simulink library "AVE_Library"  (R2025b)
settings: Solver=VariableStepAuto  StartTime=0.0  StopTime=10.0  RelTol=1e-3
undefined symbols (not defined in the file or in its folder): DiscIntNeverNeededParam
libraries: simulink x44, etargetslib x18, $bdroot x13, GenericTarget x2
(part 4 of 5)

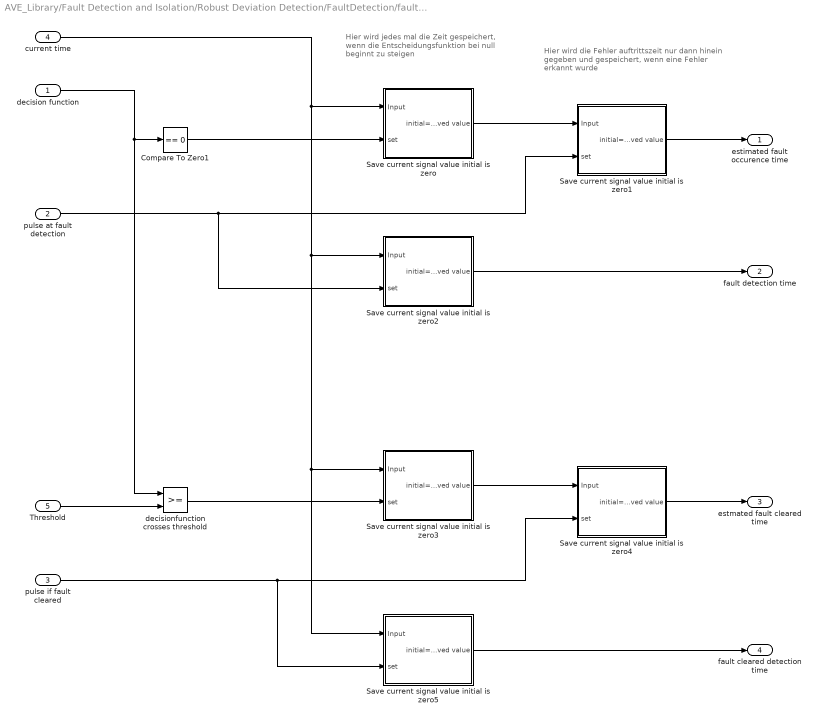
== system AVE_Library/Fault Detection and Isolation/Robust Deviation Detection/FaultDetection/fault occurence time3 ==
  note: Hier wird jedes mal die Zeit gespeichert,
      | wenn die Entscheidungsfunktion bei null
      | beginnt zu steigen
  note: Hier wird die Fehler auftrittszeit nur dann hinein
      | gegeben und gespeichert, wenn eine Fehler
      | erkannt wurde
  decision function : Inport
  pulse at fault detection : Inport  Port=2
  pulse if fault cleared : Inport  Port=3
  current time : Inport  Port=4
  Threshold : Inport  Port=5
  Compare To Zero1 : simulink/Logic and Bit Operations/Compare To Zero  relop===  OutDataTypeStr=boolean
  Save current signal value initial is zero : Subsystem  mask(save current signal value){}
      mask help:
      | If set is not zero, the input is feed throug to the output.
      | If set is zero, the output remains the last intput value when set was not zero.
      | Initial value is zero.
  Save current signal value initial is zero1 : Subsystem  mask(save current signal value){}
      mask help:
      | If set is not zero, the input is feed throug to the output.
      | If set is zero, the output remains the last intput value when set was not zero.
      | Initial value is zero.
  Save current signal value initial is zero2 : Subsystem  mask(save current signal value){}
      mask help:
      | If set is not zero, the input is feed throug to the output.
      | If set is zero, the output remains the last intput value when set was not zero.
      | Initial value is zero.
  Save current signal value initial is zero3 : Subsystem  mask(save current signal value){}
      mask help:
      | If set is not zero, the input is feed throug to the output.
      | If set is zero, the output remains the last intput value when set was not zero.
      | Initial value is zero.
  Save current signal value initial is zero4 : Subsystem  mask(save current signal value){}
      mask help:
      | If set is not zero, the input is feed throug to the output.
      | If set is zero, the output remains the last intput value when set was not zero.
      | Initial value is zero.
  Save current signal value initial is zero5 : Subsystem  mask(save current signal value){}
      mask help:
      | If set is not zero, the input is feed throug to the output.
      | If set is zero, the output remains the last intput value when set was not zero.
      | Initial value is zero.
  decisionfunction crosses threshold : RelationalOperator  OutDataTypeStr=boolean  InputSameDT=off
  estimated fault occurence time : Outport  VectorParamsAs1DForOutWhenUnconnected=off
  fault detection time : Outport  Port=2  VectorParamsAs1DForOutWhenUnconnected=off
  estmated fault cleared time : Outport  Port=3  VectorParamsAs1DForOutWhenUnconnected=off
  fault cleared detection time : Outport  Port=4  VectorParamsAs1DForOutWhenUnconnected=off
  wires:
  Compare To Zero1/1 -> Save current signal value initial is zero/2(set)
  decision function/1 -> decisionfunction crosses threshold/1, Compare To Zero1/1
  Save current signal value initial is zero1/1(initial=0  saved value) -> estimated fault occurence time/1
  pulse at fault detection/1 -> Save current signal value initial is zero2/2(set), Save current signal value initial is zero1/2(set)
  Save current signal value initial is zero/1(initial=0  saved value) -> Save current signal value initial is zero1/1(Input)
  Save current signal value initial is zero2/1(initial=0  saved value) -> fault detection time/1
  Save current signal value initial is zero3/1(initial=0  saved value) -> Save current signal value initial is zero4/1(Input)
  pulse if fault cleared/1 -> Save current signal value initial is zero5/2(set), Save current signal value initial is zero4/2(set)
  Save current signal value initial is zero4/1(initial=0  saved value) -> estmated fault cleared time/1
  current time/1 -> Save current signal value initial is zero5/1(Input), Save current signal value initial is zero3/1(Input), Save current signal value initial is zero2/1(Input), Save current signal value initial is zero/1(Input)
  decisionfunction crosses threshold/1 -> Save current signal value initial is zero3/2(set)
  Threshold/1 -> decisionfunction crosses threshold/2
  Save current signal value initial is zero5/1(initial=0  saved value) -> fault cleared detection time/1

== system AVE_Library/Fault Detection and Isolation/Robust Deviation Detection/FaultDetection/mittelwert nach oben ==
  z : Inport
  mean : Inport  Port=2
  var : Inport  Port=3
  Gain2 : Gain  Gain=0.5
  Product1 : Product  Inputs=**/  RndMeth=Zero
  Sum : Sum  Inputs=+-|
  null Vermeiden : Subsystem  mask{kleinsterWert=1e-8}
      mask prompts: kleinsterWert "Null-Mindestabstand"
      mask help:
      | Der Ausgang hält einen vorgegebenen Abstand zu Null.
      | Wenn der Eingang einen Nulldurchlauf hat, springt der Ausgang von +Mindestabstand nach -Mindestabstand, bzw. von -Mindestabstand nach +Mindestabstand. Bei Eingang ==0: Ausgang=+Mindestabstand
  log lik rat : Outport  VectorParamsAs1DForOutWhenUnconnected=off
  wires:
  null Vermeiden/1(non zero) -> Product1/3
  Gain2/1 -> Sum/2
  Sum/1 -> Product1/1
  z/1 -> Sum/1
  Product1/1 -> log lik rat/1
  var/1 -> null Vermeiden/1(value)
  mean/1 -> Gain2/1, Product1/2

== system AVE_Library/Fault Detection and Isolation/Robust Deviation Detection/FaultDetection/mittelwert nach unten ==
  z : Inport
  mean : Inport  Port=2
  var : Inport  Port=3
  Gain2 : Gain  Gain=0.5
  Product1 : Product  Inputs=**/  RndMeth=Zero
  Sum : Sum  Inputs=+-|
  null Vermeiden : Subsystem  mask{kleinsterWert=1e-8}
      mask prompts: kleinsterWert "Null-Mindestabstand"
      mask help:
      | Der Ausgang hält einen vorgegebenen Abstand zu Null.
      | Wenn der Eingang einen Nulldurchlauf hat, springt der Ausgang von +Mindestabstand nach -Mindestabstand, bzw. von -Mindestabstand nach +Mindestabstand. Bei Eingang ==0: Ausgang=+Mindestabstand
  log lik rat : Outport  VectorParamsAs1DForOutWhenUnconnected=off
  wires:
  mean/1 -> Product1/2, Gain2/1
  var/1 -> null Vermeiden/1(value)
  Product1/1 -> log lik rat/1
  z/1 -> Sum/1
  Sum/1 -> Product1/1
  Gain2/1 -> Sum/2
  null Vermeiden/1(non zero) -> Product1/3

== system AVE_Library/Fault Detection and Isolation/Robust Deviation Detection/mittelwert nach oben/null Vermeiden ==
  value : Inport
  Abs : Abs
  Constant : Constant  Value=kleinsterWert
  Gain : Gain  Gain=kleinsterWert
  Sign : Signum
  Switch : Switch  Threshold=kleinsterWert
  Switch1 : Switch  Criteria=u2 ~= 0  Threshold=1
  non zero : Outport  VectorParamsAs1DForOutWhenUnconnected=off
  wires:
  Gain/1 -> Switch1/1
  Constant/1 -> Switch1/3
  Sign/1 -> Gain/1
  Switch1/1 -> Switch/3
  Abs/1 -> Switch/2
  value/1 -> Switch/1, Sign/1, Switch1/2, Abs/1
  Switch/1 -> non zero/1

== system AVE_Library/Fault Detection and Isolation/Robust Deviation Detection/statistics/Messwertzähler ==
  measurement state : Inport
  n max : Inport  Port=2
  Constant1 : Constant  Value=0
  Memory : Memory  InheritSampleTime=on
  Saturation Dynamic : simulink/Discontinuities/Saturation Dynamic  OutMin=[]  OutMax=[]  OutDataTypeStr=Inherit: Same as second input  OutDataType=fixdt(1, 16)  OutScaling=2^-10  DoSatur=off
  Sum : Sum  Inputs=|++
  number : Outport
  wires:
  Sum/1 -> Saturation Dynamic/2
  n max/1 -> Saturation Dynamic/1
  Memory/1 -> Sum/1
  Constant1/1 -> Saturation Dynamic/3
  Saturation Dynamic/1 -> number/1, Memory/1
  measurement state/1 -> Sum/2

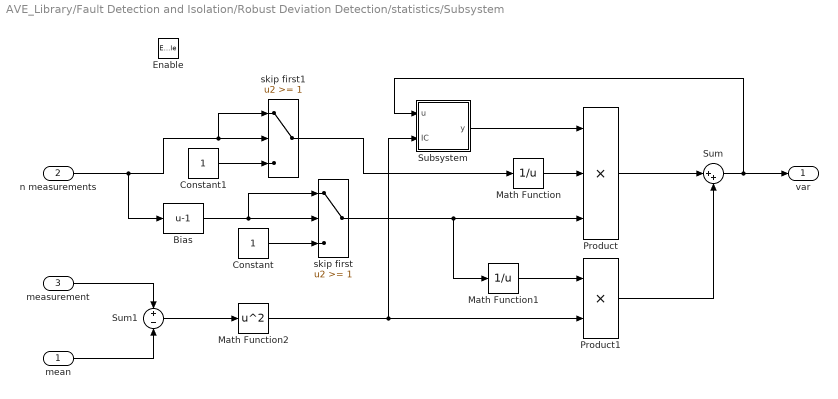
== system AVE_Library/Fault Detection and Isolation/Robust Deviation Detection/statistics/Subsystem ==
  mean : Inport
  n measurements : Inport  Port=2
  measurement : Inport  Port=3
  Enable : EnablePort
  Bias : Bias  Bias=-1  SaturateOnIntegerOverflow=off
  Constant : Constant
  Constant1 : Constant
  Math Function : Math  Operator=reciprocal  SignedPower=on
  Math Function1 : Math  Operator=reciprocal  SignedPower=on
  Math Function2 : Math  Operator=square  SignedPower=on
  Product : Product  Inputs=3  RndMeth=Zero
  Product1 : Product  RndMeth=Zero
  Subsystem : Subsystem
  Sum : Sum  Inputs=|++
  Sum1 : Sum  Inputs=+-
  skip first : Switch  Threshold=1  SaturateOnIntegerOverflow=off  InputSameDT=off
  skip first1 : Switch  Threshold=1  SaturateOnIntegerOverflow=off  InputSameDT=off
  var : Outport  InitialOutput=1
  wires:
  Product/1 -> Sum/1
  Sum/1 -> var/1, Subsystem/1(u)
  Product1/1 -> Sum/2
  Math Function/1 -> Product/2
  Bias/1 -> skip first/2, skip first/1
  Math Function1/1 -> Product1/1
  Sum1/1 -> Math Function2/1
  Math Function2/1 -> Product1/2, Subsystem/2(IC)
  n measurements/1 -> Bias/1, skip first1/1, skip first1/2
  measurement/1 -> Sum1/1
  mean/1 -> Sum1/2
  skip first/1 -> Math Function1/1, Product/3
  Subsystem/1(y) -> Product/1
  Constant/1 -> skip first/3
  skip first1/1 -> Math Function/1
  Constant1/1 -> skip first1/3

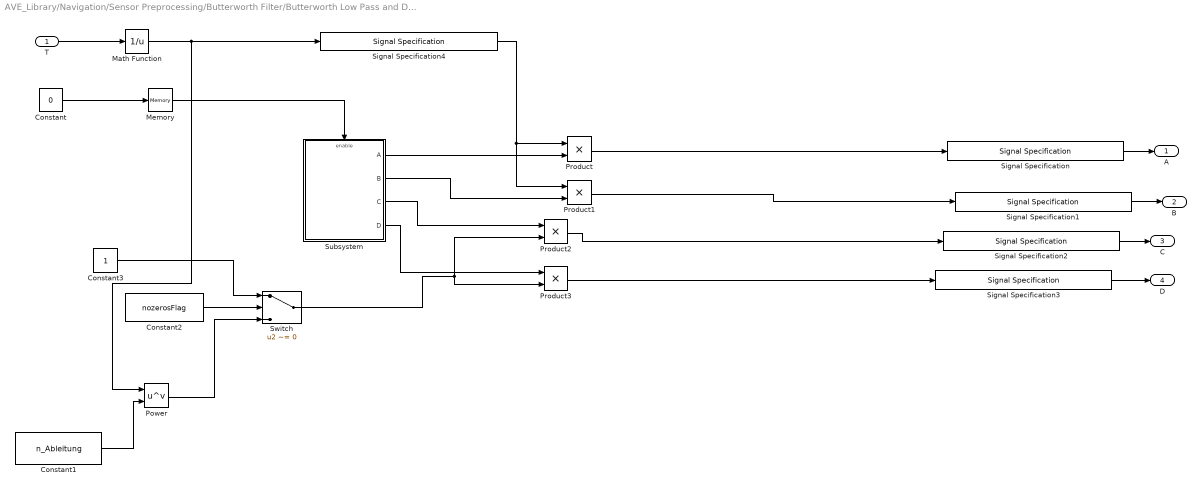
== system AVE_Library/Navigation/Sensor Preprocessing/Butterworth Filter/Butterworth Low Pass and Derivation ==
  T : Inport
  Constant : Constant  Value=0
  Constant1 : Constant  Value=n_Ableitung
  Constant2 : Constant  Value=nozerosFlag
  Constant3 : Constant
  Math Function : Math  Operator=reciprocal  SignedPower=on
  Memory : Memory  InitialCondition=1  InheritSampleTime=on
  Power : Math  Operator=pow  SignedPower=on
  Product{,1..3} (4 alike) : Product
  Signal Specification : SignalSpecification  Dimensions=[n_Ordnung_Butter_Simulink n_Ordnung_Butter_Simulink]
  Signal Specification1 : SignalSpecification  Dimensions=[n_Ordnung_Butter_Simulink 1 ]
  Signal Specification2 : SignalSpecification  Dimensions=[1 n_Ordnung_Butter_Simulink]
  Signal Specification3 : SignalSpecification  Dimensions=[1 1]
  Signal Specification4 : SignalSpecification  Dimensions=1
  Subsystem : Subsystem
  Switch : Switch  Criteria=u2 ~= 0  SaturateOnIntegerOverflow=off  InputSameDT=off
  A : Outport  VectorParamsAs1DForOutWhenUnconnected=off
  B : Outport  Port=2  VectorParamsAs1DForOutWhenUnconnected=off
  C : Outport  Port=3  VectorParamsAs1DForOutWhenUnconnected=off
  D : Outport  Port=4  VectorParamsAs1DForOutWhenUnconnected=off
  wires:
  Product1/1 -> Signal Specification1/1
  Product2/1 -> Signal Specification2/1
  Switch/1 -> Product3/2, Product2/2
  Subsystem/4(D) -> Product3/1
  Subsystem/3(C) -> Product2/1
  Product3/1 -> Signal Specification3/1
  Constant2/1 -> Switch/2
  Power/1 -> Switch/3
  Constant1/1 -> Power/2
  Math Function/1 -> Power/1, Signal Specification4/1
  Constant3/1 -> Switch/1
  Memory/1 -> Subsystem/Enable
  Signal Specification4/1 -> Product1/1, Product/1
  Constant/1 -> Memory/1
  Product/1 -> Signal Specification/1
  Subsystem/2(B) -> Product1/2
  Subsystem/1(A) -> Product/2
  T/1 -> Math Function/1
  Signal Specification/1 -> A/1
  Signal Specification1/1 -> B/1
  Signal Specification2/1 -> C/1
  Signal Specification3/1 -> D/1

== system AVE_Library/Navigation/Sensor Preprocessing/Butterworth Filter/Zustandsraummodell x0=x_t_inf(u=u_t_0) ==
  A : Inport
  B : Inport  Port=2
  C : Inport  Port=3
  D : Inport  Port=4
  u : Inport  Port=5  Partition=on  PartitionDimension=1  PartitionWidth=1  PartitionOffset=0
  reset : Inport  Port=6
  Divide : Product  Inputs=/**  Multiplication=Matrix(*)
  For Each : ForEach  DisableCoverage=on
  Gain : Gain  Gain=-1
      settings: AttributesFormatString== -1
  Terminator : Terminator
  Zustandsraummodell discrete Integrator : Subsystem
  y : Outport  ConcatenationDimension=1  VectorParamsAs1DForOutWhenUnconnected=off
  wires:
  reset/1 -> Zustandsraummodell discrete Integrator/7(reset)
  Gain/1 -> Zustandsraummodell discrete Integrator/6(y_ini)
  C/1 -> Zustandsraummodell discrete Integrator/3(C)
  B/1 -> Zustandsraummodell discrete Integrator/2(B), Divide/2
  D/1 -> Zustandsraummodell discrete Integrator/4(D)
  Zustandsraummodell discrete Integrator/1(y) -> y/1
  A/1 -> Zustandsraummodell discrete Integrator/1(A), Divide/1
  Divide/1 -> Gain/1
  u/1 -> Zustandsraummodell discrete Integrator/5(u), Divide/3
  Zustandsraummodell discrete Integrator/2(x) -> Terminator/1

== system AVE_Library/Fault Detection and Isolation/Robust Deviation Detection/FaultDetection/Threshold evaluation1/FehlerSpeicher ==
  Input : Inport
  set : Inport  Port=2
  Init : Switch  Criteria=u2 ~= 0  OutDataTypeStr=Inherit: Inherit via back propagation  ZeroCross=off  SaturateOnIntegerOverflow=off  InputSameDT=off
  Memory : Memory  InheritSampleTime=on
  Reset : Switch  Criteria=u2 ~= 0  OutDataTypeStr=Inherit: Inherit via back propagation  ZeroCross=off  SaturateOnIntegerOverflow=off  InputSameDT=off
  initial=0  saved value : Outport  VectorParamsAs1DForOutWhenUnconnected=off
  wires:
  Input/1 -> Init/1, Reset/1
  Reset/1 -> Memory/1
  Init/1 -> Reset/3, initial=0  saved value/1
  Memory/1 -> Init/3
  set/1 -> Init/2, Reset/2

== system AVE_Library/Fault Detection and Isolation/Robust Deviation Detection/FaultDetection/Threshold evaluation3/FehlerSpeicher ==
  Input : Inport
  set : Inport  Port=2
  Init : Switch  Criteria=u2 ~= 0  OutDataTypeStr=Inherit: Inherit via back propagation  ZeroCross=off  SaturateOnIntegerOverflow=off  InputSameDT=off
  Memory : Memory  InheritSampleTime=on
  Reset : Switch  Criteria=u2 ~= 0  OutDataTypeStr=Inherit: Inherit via back propagation  ZeroCross=off  SaturateOnIntegerOverflow=off  InputSameDT=off
  initial=0  saved value : Outport  VectorParamsAs1DForOutWhenUnconnected=off
  wires:
  set/1 -> Reset/2, Init/2
  Memory/1 -> Init/3
  Init/1 -> initial=0  saved value/1, Reset/3
  Reset/1 -> Memory/1
  Input/1 -> Reset/1, Init/1

== system AVE_Library/Fault Detection and Isolation/Robust Deviation Detection/FaultDetection/Worst Time/Save current signal value initial is zero ==
  Input : Inport
  set : Inport  Port=2
  Init : Switch  Criteria=u2 ~= 0  OutDataTypeStr=Inherit: Inherit via back propagation  ZeroCross=off  SaturateOnIntegerOverflow=off  InputSameDT=off
  Memory : Memory  InheritSampleTime=on
  Reset : Switch  Criteria=u2 ~= 0  OutDataTypeStr=Inherit: Inherit via back propagation  ZeroCross=off  SaturateOnIntegerOverflow=off  InputSameDT=off
  initial=0  saved value : Outport  VectorParamsAs1DForOutWhenUnconnected=off
  wires:
  set/1 -> Reset/2, Init/2
  Memory/1 -> Init/3
  Init/1 -> initial=0  saved value/1, Reset/3
  Reset/1 -> Memory/1
  Input/1 -> Reset/1, Init/1

== system AVE_Library/Fault Detection and Isolation/Robust Deviation Detection/FaultDetection/Worst Time/Save current signal value initial is zero2 ==
  Input : Inport
  set : Inport  Port=2
  Init : Switch  Criteria=u2 ~= 0  OutDataTypeStr=Inherit: Inherit via back propagation  ZeroCross=off  SaturateOnIntegerOverflow=off  InputSameDT=off
  Memory : Memory  InheritSampleTime=on
  Reset : Switch  Criteria=u2 ~= 0  OutDataTypeStr=Inherit: Inherit via back propagation  ZeroCross=off  SaturateOnIntegerOverflow=off  InputSameDT=off
  initial=0  saved value : Outport  VectorParamsAs1DForOutWhenUnconnected=off
  wires:
  Input/1 -> Init/1, Reset/1
  Reset/1 -> Memory/1
  Init/1 -> Reset/3, initial=0  saved value/1
  Memory/1 -> Init/3
  set/1 -> Init/2, Reset/2

== system AVE_Library/Fault Detection and Isolation/Robust Deviation Detection/FaultDetection/fault occurence time1/Save current signal value initial is zero ==
  Input : Inport
  set : Inport  Port=2
  Init : Switch  Criteria=u2 ~= 0  OutDataTypeStr=Inherit: Inherit via back propagation  ZeroCross=off  SaturateOnIntegerOverflow=off  InputSameDT=off
  Memory : Memory  InheritSampleTime=on
  Reset : Switch  Criteria=u2 ~= 0  OutDataTypeStr=Inherit: Inherit via back propagation  ZeroCross=off  SaturateOnIntegerOverflow=off  InputSameDT=off
  initial=0  saved value : Outport  VectorParamsAs1DForOutWhenUnconnected=off
  wires:
  Input/1 -> Init/1, Reset/1
  Reset/1 -> Memory/1
  Init/1 -> Reset/3, initial=0  saved value/1
  Memory/1 -> Init/3
  set/1 -> Init/2, Reset/2

== system AVE_Library/Fault Detection and Isolation/Robust Deviation Detection/FaultDetection/fault occurence time1/Save current signal value initial is zero1 ==
  Input : Inport
  set : Inport  Port=2
  Init : Switch  Criteria=u2 ~= 0  OutDataTypeStr=Inherit: Inherit via back propagation  ZeroCross=off  SaturateOnIntegerOverflow=off  InputSameDT=off
  Memory : Memory  InheritSampleTime=on
  Reset : Switch  Criteria=u2 ~= 0  OutDataTypeStr=Inherit: Inherit via back propagation  ZeroCross=off  SaturateOnIntegerOverflow=off  InputSameDT=off
  initial=0  saved value : Outport  VectorParamsAs1DForOutWhenUnconnected=off
  wires:
  Input/1 -> Init/1, Reset/1
  Reset/1 -> Memory/1
  Init/1 -> Reset/3, initial=0  saved value/1
  Memory/1 -> Init/3
  set/1 -> Init/2, Reset/2

== system AVE_Library/Fault Detection and Isolation/Robust Deviation Detection/FaultDetection/fault occurence time1/Save current signal value initial is zero2 ==
  Input : Inport
  set : Inport  Port=2
  Init : Switch  Criteria=u2 ~= 0  OutDataTypeStr=Inherit: Inherit via back propagation  ZeroCross=off  SaturateOnIntegerOverflow=off  InputSameDT=off
  Memory : Memory  InheritSampleTime=on
  Reset : Switch  Criteria=u2 ~= 0  OutDataTypeStr=Inherit: Inherit via back propagation  ZeroCross=off  SaturateOnIntegerOverflow=off  InputSameDT=off
  initial=0  saved value : Outport  VectorParamsAs1DForOutWhenUnconnected=off
  wires:
  set/1 -> Reset/2, Init/2
  Memory/1 -> Init/3
  Init/1 -> initial=0  saved value/1, Reset/3
  Reset/1 -> Memory/1
  Input/1 -> Reset/1, Init/1

== system AVE_Library/Fault Detection and Isolation/Robust Deviation Detection/FaultDetection/fault occurence time1/Save current signal value initial is zero3 ==
  Input : Inport
  set : Inport  Port=2
  Init : Switch  Criteria=u2 ~= 0  OutDataTypeStr=Inherit: Inherit via back propagation  ZeroCross=off  SaturateOnIntegerOverflow=off  InputSameDT=off
  Memory : Memory  InheritSampleTime=on
  Reset : Switch  Criteria=u2 ~= 0  OutDataTypeStr=Inherit: Inherit via back propagation  ZeroCross=off  SaturateOnIntegerOverflow=off  InputSameDT=off
  initial=0  saved value : Outport  VectorParamsAs1DForOutWhenUnconnected=off
  wires:
  set/1 -> Reset/2, Init/2
  Memory/1 -> Init/3
  Init/1 -> initial=0  saved value/1, Reset/3
  Reset/1 -> Memory/1
  Input/1 -> Reset/1, Init/1

== system AVE_Library/Fault Detection and Isolation/Robust Deviation Detection/FaultDetection/fault occurence time1/Save current signal value initial is zero4 ==
  Input : Inport
  set : Inport  Port=2
  Init : Switch  Criteria=u2 ~= 0  OutDataTypeStr=Inherit: Inherit via back propagation  ZeroCross=off  SaturateOnIntegerOverflow=off  InputSameDT=off
  Memory : Memory  InheritSampleTime=on
  Reset : Switch  Criteria=u2 ~= 0  OutDataTypeStr=Inherit: Inherit via back propagation  ZeroCross=off  SaturateOnIntegerOverflow=off  InputSameDT=off
  initial=0  saved value : Outport  VectorParamsAs1DForOutWhenUnconnected=off
  wires:
  set/1 -> Reset/2, Init/2
  Memory/1 -> Init/3
  Init/1 -> initial=0  saved value/1, Reset/3
  Reset/1 -> Memory/1
  Input/1 -> Reset/1, Init/1

== system AVE_Library/Fault Detection and Isolation/Robust Deviation Detection/FaultDetection/fault occurence time1/Save current signal value initial is zero5 ==
  Input : Inport
  set : Inport  Port=2
  Init : Switch  Criteria=u2 ~= 0  OutDataTypeStr=Inherit: Inherit via back propagation  ZeroCross=off  SaturateOnIntegerOverflow=off  InputSameDT=off
  Memory : Memory  InheritSampleTime=on
  Reset : Switch  Criteria=u2 ~= 0  OutDataTypeStr=Inherit: Inherit via back propagation  ZeroCross=off  SaturateOnIntegerOverflow=off  InputSameDT=off
  initial=0  saved value : Outport  VectorParamsAs1DForOutWhenUnconnected=off
  wires:
  Input/1 -> Init/1, Reset/1
  Reset/1 -> Memory/1
  Init/1 -> Reset/3, initial=0  saved value/1
  Memory/1 -> Init/3
  set/1 -> Init/2, Reset/2

== system AVE_Library/Fault Detection and Isolation/Robust Deviation Detection/FaultDetection/fault occurence time3/Save current signal value initial is zero ==
  Input : Inport
  set : Inport  Port=2
  Init : Switch  Criteria=u2 ~= 0  OutDataTypeStr=Inherit: Inherit via back propagation  ZeroCross=off  SaturateOnIntegerOverflow=off  InputSameDT=off
  Memory : Memory  InheritSampleTime=on
  Reset : Switch  Criteria=u2 ~= 0  OutDataTypeStr=Inherit: Inherit via back propagation  ZeroCross=off  SaturateOnIntegerOverflow=off  InputSameDT=off
  initial=0  saved value : Outport  VectorParamsAs1DForOutWhenUnconnected=off
  wires:
  set/1 -> Reset/2, Init/2
  Memory/1 -> Init/3
  Init/1 -> initial=0  saved value/1, Reset/3
  Reset/1 -> Memory/1
  Input/1 -> Reset/1, Init/1

== system AVE_Library/Fault Detection and Isolation/Robust Deviation Detection/FaultDetection/fault occurence time3/Save current signal value initial is zero1 ==
  Input : Inport
  set : Inport  Port=2
  Init : Switch  Criteria=u2 ~= 0  OutDataTypeStr=Inherit: Inherit via back propagation  ZeroCross=off  SaturateOnIntegerOverflow=off  InputSameDT=off
  Memory : Memory  InheritSampleTime=on
  Reset : Switch  Criteria=u2 ~= 0  OutDataTypeStr=Inherit: Inherit via back propagation  ZeroCross=off  SaturateOnIntegerOverflow=off  InputSameDT=off
  initial=0  saved value : Outport  VectorParamsAs1DForOutWhenUnconnected=off
  wires:
  set/1 -> Reset/2, Init/2
  Memory/1 -> Init/3
  Init/1 -> initial=0  saved value/1, Reset/3
  Reset/1 -> Memory/1
  Input/1 -> Reset/1, Init/1

== system AVE_Library/Fault Detection and Isolation/Robust Deviation Detection/FaultDetection/fault occurence time3/Save current signal value initial is zero2 ==
  Input : Inport
  set : Inport  Port=2
  Init : Switch  Criteria=u2 ~= 0  OutDataTypeStr=Inherit: Inherit via back propagation  ZeroCross=off  SaturateOnIntegerOverflow=off  InputSameDT=off
  Memory : Memory  InheritSampleTime=on
  Reset : Switch  Criteria=u2 ~= 0  OutDataTypeStr=Inherit: Inherit via back propagation  ZeroCross=off  SaturateOnIntegerOverflow=off  InputSameDT=off
  initial=0  saved value : Outport  VectorParamsAs1DForOutWhenUnconnected=off
  wires:
  Input/1 -> Init/1, Reset/1
  Reset/1 -> Memory/1
  Init/1 -> Reset/3, initial=0  saved value/1
  Memory/1 -> Init/3
  set/1 -> Init/2, Reset/2

== system AVE_Library/Fault Detection and Isolation/Robust Deviation Detection/FaultDetection/fault occurence time3/Save current signal value initial is zero3 ==
  Input : Inport
  set : Inport  Port=2
  Init : Switch  Criteria=u2 ~= 0  OutDataTypeStr=Inherit: Inherit via back propagation  ZeroCross=off  SaturateOnIntegerOverflow=off  InputSameDT=off
  Memory : Memory  InheritSampleTime=on
  Reset : Switch  Criteria=u2 ~= 0  OutDataTypeStr=Inherit: Inherit via back propagation  ZeroCross=off  SaturateOnIntegerOverflow=off  InputSameDT=off
  initial=0  saved value : Outport  VectorParamsAs1DForOutWhenUnconnected=off
  wires:
  Input/1 -> Init/1, Reset/1
  Reset/1 -> Memory/1
  Init/1 -> Reset/3, initial=0  saved value/1
  Memory/1 -> Init/3
  set/1 -> Init/2, Reset/2

== system AVE_Library/Fault Detection and Isolation/Robust Deviation Detection/FaultDetection/fault occurence time3/Save current signal value initial is zero4 ==
  Input : Inport
  set : Inport  Port=2
  Init : Switch  Criteria=u2 ~= 0  OutDataTypeStr=Inherit: Inherit via back propagation  ZeroCross=off  SaturateOnIntegerOverflow=off  InputSameDT=off
  Memory : Memory  InheritSampleTime=on
  Reset : Switch  Criteria=u2 ~= 0  OutDataTypeStr=Inherit: Inherit via back propagation  ZeroCross=off  SaturateOnIntegerOverflow=off  InputSameDT=off
  initial=0  saved value : Outport  VectorParamsAs1DForOutWhenUnconnected=off
  wires:
  Input/1 -> Init/1, Reset/1
  Reset/1 -> Memory/1
  Init/1 -> Reset/3, initial=0  saved value/1
  Memory/1 -> Init/3
  set/1 -> Init/2, Reset/2

== system AVE_Library/Fault Detection and Isolation/Robust Deviation Detection/FaultDetection/fault occurence time3/Save current signal value initial is zero5 ==
  Input : Inport
  set : Inport  Port=2
  Init : Switch  Criteria=u2 ~= 0  OutDataTypeStr=Inherit: Inherit via back propagation  ZeroCross=off  SaturateOnIntegerOverflow=off  InputSameDT=off
  Memory : Memory  InheritSampleTime=on
  Reset : Switch  Criteria=u2 ~= 0  OutDataTypeStr=Inherit: Inherit via back propagation  ZeroCross=off  SaturateOnIntegerOverflow=off  InputSameDT=off
  initial=0  saved value : Outport  VectorParamsAs1DForOutWhenUnconnected=off
  wires:
  set/1 -> Reset/2, Init/2
  Memory/1 -> Init/3
  Init/1 -> initial=0  saved value/1, Reset/3
  Reset/1 -> Memory/1
  Input/1 -> Reset/1, Init/1

== system AVE_Library/Fault Detection and Isolation/Robust Deviation Detection/FaultDetection/mittelwert nach oben/null Vermeiden ==
  value : Inport
  Abs : Abs
  Constant : Constant  Value=kleinsterWert
  Gain : Gain  Gain=kleinsterWert
  Sign : Signum
  Switch : Switch  Threshold=kleinsterWert
  Switch1 : Switch  Criteria=u2 ~= 0  Threshold=1
  non zero : Outport  VectorParamsAs1DForOutWhenUnconnected=off
  wires:
  Gain/1 -> Switch1/1
  Constant/1 -> Switch1/3
  Sign/1 -> Gain/1
  Switch1/1 -> Switch/3
  Abs/1 -> Switch/2
  value/1 -> Switch/1, Sign/1, Switch1/2, Abs/1
  Switch/1 -> non zero/1

== system AVE_Library/Fault Detection and Isolation/Robust Deviation Detection/FaultDetection/mittelwert nach unten/null Vermeiden ==
  value : Inport
  Abs : Abs
  Constant : Constant  Value=kleinsterWert
  Gain : Gain  Gain=kleinsterWert
  Sign : Signum
  Switch : Switch  Threshold=kleinsterWert
  Switch1 : Switch  Criteria=u2 ~= 0  Threshold=1
  non zero : Outport  VectorParamsAs1DForOutWhenUnconnected=off
  wires:
  Switch/1 -> non zero/1
  value/1 -> Abs/1, Switch1/2, Sign/1, Switch/1
  Abs/1 -> Switch/2
  Switch1/1 -> Switch/3
  Sign/1 -> Gain/1
  Constant/1 -> Switch1/3
  Gain/1 -> Switch1/1

== system AVE_Library/Fault Detection and Isolation/Robust Deviation Detection/statistics/Subsystem/Subsystem ==
  note: Xnew
  note: Initial Value
  u : Inport
  IC : Inport  Port=2
  FixPt Data Type Duplicate1 : DataTypeDuplicate  NumInputPorts=3
  Gain : Gain  Gain=0
  Init : Switch  Criteria=u2 ~= 0  OutDataTypeStr=Inherit: Inherit via back propagation  ZeroCross=off  SaturateOnIntegerOverflow=off  InputSameDT=off
  Memory : Memory  InitialCondition=1  InheritSampleTime=on
  Memory1 : Memory  InheritSampleTime=on
  y : Outport
  wires:
  Memory1/1 -> Init/3  "Xold"
  Init/1 -> y/1, FixPt Data Type Duplicate1/1
  IC/1 -> Init/1, FixPt Data Type Duplicate1/3
  Gain/1 -> Memory/1
  Memory/1 -> Init/2
  u/1 -> FixPt Data Type Duplicate1/2, Memory1/1, Gain/1

== system AVE_Library/Navigation/Sensor Preprocessing/Butterworth Filter/Butterworth Low Pass and Derivation/Subsystem ==
  Enable : EnablePort
  Butter 2 p,k1 : MATLAB Function  TreatAsAtomicUnit=on
  Constant : Constant  Value=Nullstellen
  myzp2ss : MATLAB Function  TreatAsAtomicUnit=on
  A : Outport  VectorParamsAs1DForOutWhenUnconnected=off
  B : Outport  Port=2  VectorParamsAs1DForOutWhenUnconnected=off
  C : Outport  Port=3  VectorParamsAs1DForOutWhenUnconnected=off
  D : Outport  Port=4  VectorParamsAs1DForOutWhenUnconnected=off
  wires:
  Butter 2 p,k1/1(p) -> myzp2ss/2(p)
  Constant/1 -> myzp2ss/1(z)
  myzp2ss/1(a) -> A/1
  myzp2ss/4(d) -> D/1
  myzp2ss/3(c) -> C/1
  myzp2ss/2(b) -> B/1

== system AVE_Library/Navigation/Sensor Preprocessing/Butterworth Filter/Zustandsraummodell x0=x_t_inf(u=u_t_0)/Zustandsraummodell discrete Integrator ==
  A : Inport
  B : Inport  Port=2
  C : Inport  Port=3
  D : Inport  Port=4
  u : Inport  Port=5
  y_ini : Inport  Port=6
  reset : Inport  Port=7
  Discrete-Time Integrator : DiscreteIntegrator  ExternalReset=level  InitialConditionSource=external  SampleTime=-1  ICPrevOutput=DiscIntNeverNeededParam  ICPrevScaledInput=DiscIntNeverNeededParam
  Product{,1..3} (4 alike) : Product  Multiplication=Matrix(*)
  Reshape : Reshape  OutputDimensionality=Column vector (2-D)
  Sum : Sum  Inputs=|++
  Sum1 : Sum  Inputs=++|
  y : Outport  VectorParamsAs1DForOutWhenUnconnected=off
  x : Outport  Port=2  VectorParamsAs1DForOutWhenUnconnected=off
  wires:
  y_ini/1 -> Reshape/1
  Discrete-Time Integrator/1 -> Product/2, x/1, Product2/2
  A/1 -> Product/1
  Sum/1 -> Discrete-Time Integrator/1
  Product1/1 -> Sum/1
  B/1 -> Product1/1
  Product/1 -> Sum/2
  C/1 -> Product2/1
  Sum1/1 -> y/1
  Product2/1 -> Sum1/2
  D/1 -> Product3/1
  Product3/1 -> Sum1/1
  u/1 -> Product3/2, Product1/2
  Reshape/1 -> Discrete-Time Integrator/3
  reset/1 -> Discrete-Time Integrator/2

== matlab function AVE_Library/Essential/Transformation/Transform Sensor Velocity UVW/MATLAB Function ==
  data: uSensor input; uBody output; vSensor input; wSensor input; R_b2s input; r_b2s input; pqr input; vBody output; wBody output
function [uBody, vBody, wBody] = VelocityUVW_Sensor2Body(uSensor, vSensor, wSensor, R_b2s, r_b2s, pqr)
    [uBody, vBody, wBody] = ave.TransformSensor2BodyVelocityUVW(uSensor, vSensor, wSensor, R_b2s, r_b2s, pqr);
end

== matlab function AVE_Library/Essential/Transformation/Euler ZYX To Rotation Matrix/MATLAB Function ==
  data: roll input; R output; pitch input; yaw input
function R = Rb2n(roll, pitch, yaw)
    R = eul2rotm([yaw, pitch, roll]);
end

== matlab function AVE_Library/Essential/Signal Logics/Toggle Value Up Down/MATLAB Function ==
  data: up input boolean size=1; y output uint8 size=1; down input boolean size=1; maxValue parameter uint8 size=1
function y = ToggleUpDown(up, down, maxValue)
    persistent value;
    if(isempty(value)), value = int32(0); end
    if(up), value = value + int32(1); end
    if(down), value = value - int32(1); end
    if(value < int32(0)), value = int32(0); end
    if(value > int32(maxValue)), value = int32(maxValue); end
    y = uint8(value);
end

== matlab function AVE_Library/Essential/Signal Logics/Index Of Latest Trigger/MATLAB Function ==
  data: buttons input; value output
function value = fcn(buttons)
    persistent v;
    if(isempty(v)), v = uint8(0); end
    idx = find(buttons, 1);
    if(~isempty(idx))
        v = uint8(idx(1) - 1);
    end
    value = v;
end

== matlab function AVE_Library/Essential/Is Finite/MATLAB Function ==
  data: u input; y output
function y = IsFinite(u)
    y = isfinite(u);
end

== matlab function AVE_Library/Essential/Contains NaN/MATLAB Function ==
  data: u input; y output
function y = ContainsNaN(u)
    y = any(isnan(u), 'all');
end

== matlab function AVE_Library/Essential/Signal Logics/Resetable Toggle Value Up/MATLAB Function ==
  data: triggerRise input boolean size=1; value output uint8 size=1; reset input boolean size=1; maxValue parameter uint8 size=1
function value = ResetableToggle(triggerRise, reset, maxValue)
    persistent out;
    if(isempty(out) || reset)
        out = uint8(0);
    elseif(triggerRise)
        out = out + uint8(1);
        if(out > maxValue)
            out = uint8(0);
        end
    end
    value = out;
end

== matlab function AVE_Library/Essential/Transformation/Yaw To Rotation Matrix/MATLAB Function ==
  data: R output; yaw input
function R = Rb2n(yaw)
    c3 = cos(yaw);
    s3 = sin(yaw);
    R = [c3 -s3; s3 c3];
end

== matlab function AVE_Library/Essential/Signal Logics/Resetable Index Of Latest Trigger/MATLAB Function ==
  data: buttons input; value output; reset input; resetValue input
function value = fcn(buttons,reset,resetValue)
    persistent v;
    if(isempty(v) || reset), v = uint8(resetValue); end
    idx = find(buttons, 1);
    if(~isempty(idx))
        v = uint8(idx(1) - 1);
    end
    value = v;
end

== matlab function AVE_Library/Essential/Transformation/Transform Sensor Quaternion WXYZ/MATLAB Function ==
  data: quaternionSensor input double size=4; quaternionBody output double size=4; R_b2s input double size=[3 3]
function quaternionBody = QuaternionWXYZ_Sensor2Body(quaternionSensor, R_b2s)
    quaternionBody = ave.TransformSensor2BodyQuaternionWXYZ(quaternionSensor, R_b2s);
end

== matlab function AVE_Library/Essential/Equations of Motion/Kinematic 6DoF Geographic/MATLAB Function ==
  data: phi input; lat output; lambda input; lon output
function [lat, lon] = EnsureLatLonRange(phi, lambda)
    %EnsureLatLonRange Convert phi [rad] and lambda [rad] to latitude [rad] and longitude [rad] with latitude being in range [-pi/2, +pi/2] and longitude being in range [-pi; +pi).
    % 
    % PARAMETERS
    % phi    ... Input angle for latitude in radians.
    % lambda ... Input angle for longitude in radians.
    % 
    % RETURN
    % lat ... Output angle for latitude [rad] being in range [-pi/2, +pi/2].
    % lon ... Output angle for longitude [rad] being in range [-pi, +pi).
    const_pi_half = 0.5 * pi;
    const_pi_2 = (pi + pi);

    % Make sure that inputs are scalars
    assert(isscalar(phi), 'Input "phi" must be scalar!');
    assert(isscalar(lambda), 'Input "lambda" must be scalar!');

    % Convert phi to symmetric angle [-pi, pi)
    phi = double(mod(phi, const_pi_2));
    phi = phi - double(phi >= pi) * const_pi_2;

    % Check for (phi > pi/2) and (phi < -pi/2)
    if(phi > const_pi_half)
        phi = pi - phi;
        lambda = lambda + pi;
    elseif(phi < -const_pi_half)
        phi = -pi - phi;
        lambda = lambda + pi;
    end

    % Convert lambda to symmetric angle [-pi, pi)
    lambda = double(mod(lambda, const_pi_2));
    lambda = lambda - double(lambda >= pi) * const_pi_2;

    % Set output
    lat = phi;
    lon = lambda;
end

== matlab function AVE_Library/Essential/SHA256/SHA256 ==
  data: bytes input uint8; hash output uint8 size=32; numBytes input
function hash = ComputeSHA256(bytes, numBytes)
    hash = ave.sha256(bytes, numBytes);
end

== matlab function AVE_Library/Essential/Signal Logics/Hold Timeout/MATLAB Function ==
  data: time input; tfHoldTimeout output; tfTimeout input; timeHold input
function tfHoldTimeout = HoldTimeout(time, tfTimeout, timeHold)
    persistent timeOfTimeout;
    persistent prevTimeout;
    if(isempty(timeOfTimeout)), timeOfTimeout = -2*timeHold; end
    if(isempty(prevTimeout)), prevTimeout = true; end

    % Detect new timeout
    if((tfTimeout && ~prevTimeout) && (time - timeOfTimeout >= timeHold))
        timeOfTimeout = time;
    end
    prevTimeout = tfTimeout;

    % Hold timeout for at least
    tfHoldTimeout = (time - timeOfTimeout <= timeHold) || tfTimeout;
end

== matlab function AVE_Library/Essential/Symmetrical Angle/MATLAB Function1 ==
  data: u input; y output
function y = SA(u)
    y = ave.SymmetricalAngle(u);
end

== matlab function AVE_Library/Guidance/Trajectory Track Error/MATLAB Function1 ==
  data: valid output boolean size=1; trackError output double size=2; time input double size=1; positionLLA input double size=3; matTimeLatLon input double; numPoints input int32 size=1; closestSegmentIndices output int32 size=2; closestSegmentLinearInterpolationRatio output double size=1; targetSegmentIndices output int32 size=2; targetSegmentLinearInterpolationRatio output double size=1
function [valid, trackError, closestSegmentIndices, closestSegmentLinearInterpolationRatio, targetSegmentIndices, targetSegmentLinearInterpolationRatio] = TrajectoryTrackError(time, positionLLA, matTimeLatLon, numPoints)
    [valid, trackError, closestSegmentIndices, closestSegmentLinearInterpolationRatio, targetSegmentIndices, targetSegmentLinearInterpolationRatio] = ave.TrajectoryTrackError(time, positionLLA, matTimeLatLon, numPoints);
end

== matlab function AVE_Library/Essential/Equations of Motion/Strapdown Algorithm/MATLAB Function ==
  data: sampletime input double size=1; outPositionLLA output double size=3; imuAcceleration input double size=3; imuAngularRate input double size=3; positionLLA input double size=3; orientationQuaternionWXYZ input double size=4; velocityUVW input double size=3; outOrientationQuaternionWXYZ output double size=4; outVelocityUVW output double size=3
function [outPositionLLA, outOrientationQuaternionWXYZ, outVelocityUVW] = StrapdownAlgorithm(sampletime, imuAcceleration, imuAngularRate, positionLLA, orientationQuaternionWXYZ, velocityUVW)
    [outPositionLLA, outOrientationQuaternionWXYZ, outVelocityUVW] = ave.StrapdownAlgorithm(sampletime, imuAcceleration, imuAngularRate, positionLLA, orientationQuaternionWXYZ, velocityUVW);
end

== matlab function AVE_Library/Navigation/Sensor Preprocessing/Smoothed Quaternion Time Derivative/SmoothedOrientationDeviation ==
  data: time input double size=1; trigger input boolean size=1; p output double size=1; qw input double size=1; qx input double size=1; qy input double size=1; qz input double size=1; q output double size=1; r output double size=1; T input double size=1
function [p,q,r] = SmoothedOrientationDeviation(time,trigger,qw,qx,qy,qz,T)
    persistent pqr;
    if(isempty(pqr)), pqr = [0.0;0.0;0.0]; end
    persistent prevTime;
    if(isempty(prevTime)), prevTime = time; end
    persistent qFiltered;
    if(isempty(qFiltered) && trigger), qFiltered = [qw;qx;qy;qz]; end
    persistent prevQInput;
    if(isempty(prevQInput) && trigger), prevQInput = [qw;qx;qy;qz]; end
    persistent prevQFiltered;
    if(isempty(prevQFiltered) && trigger), prevQFiltered = [qw;qx;qy;qz]; end

    % Only update angular velocity if new quaternion measurement is available
    dt = time - prevTime;
    if(trigger && (dt > 0.0) && ~isempty(qFiltered) && ~isempty(prevQInput) && ~isempty(prevQFiltered))
        prevTime = time;

        % Input quaternion
        qin = [qw;qx;qy;qz];
        L = norm(qin);
        if(L > 0)
            qin = qin / L;
        else
            qin = [1;0;0;0];
        end

        % Low pass filtering for input quaternion
        T = max(0,T);
        s1 = (T+T - dt) / (T+T + dt);
        s2 = dt / (T+T + dt);
        qFiltered = s1 * qFiltered + s2 * (qin + prevQInput);
        prevQInput = qin;

        % Normalize filtered quaternion
        qFiltered = qFiltered / norm(qFiltered);

        % Time derivative of quaternion
        qdot = (qFiltered - prevQFiltered) / dt;
        prevQFiltered = qFiltered;

        % Update angular rate
        qw = qFiltered(1);
        qx = qFiltered(2);
        qy = qFiltered(3);
        qz = qFiltered(4);
        Q = 0.5 * [-qx -qy -qz; qw -qz qy; qz qw -qx; -qy qx qw];
        pqr = pinv(Q) * qdot;
    end

    % Set output
    p = pqr(1);
    q = pqr(2);
    r = pqr(3);
end

== matlab function AVE_Library/Navigation/Sensor Preprocessing/Triggered Low Pass/TriggeredLowPass ==
  data: time input double size=1; trigger input boolean size=1; y output double; u input double; T input double size=1
function y = TriggeredLowPass(time,trigger,u,T)
    persistent prevTime;
    if(isempty(prevTime)), prevTime = time; end
    persistent prevY;
    if(isempty(prevY) && trigger), prevY = u; end
    persistent prevU;
    if(isempty(prevU) && trigger), prevU = u; end

    % Only update if new measurement is available
    dt = time - prevTime;
    if(trigger && (dt > 0.0) && ~isempty(prevY) && ~isempty(prevU))
        prevTime = time;
        T = max(0,T);
        s1 = (T+T - dt) / (T+T + dt);
        s2 = dt / (T+T + dt);
        prevY = s1 * prevY + s2 * (u + prevU);
        prevU = u;
    end

    % Set output
    y = u;
    if(~isempty(prevY)), y = prevY; end
end

== matlab function AVE_Library/Navigation/Sensor Preprocessing/Detect Outliers 1D/MATLAB Function ==
  data: triggerNewData input boolean size=1; data input double size=1; numberOfOutliers output uint32 size=1; threshold input double size=1; maxNumOutliers input uint32 size=1
function numberOfOutliers = DetectOutlier(triggerNewData, data, threshold, maxNumOutliers)
    persistent prevData; if(isempty(prevData)), prevData = data; end
    persistent numOutliers; if(isempty(numOutliers)), numOutliers = uint32(0); end

    % New data must be available
    if(uint8(triggerNewData))
        % Check whether the new data indicates an outlier
        outlier = abs(data - prevData) >= abs(threshold);

        % If it's an outlier, increment the counter
        % If not, save new previous value and reset counter
        if(outlier)
            % If the maximum number of outliers is exceeded, then ignore the outlier and assume it as a valid value
            if(numOutliers >= uint32(maxNumOutliers))
                prevData = data;
                numOutliers = uint32(0);
            else
                numOutliers = numOutliers + uint32(1);
            end
        else
            prevData = data;
            numOutliers = uint32(0);
        end
    end

    % Set output
    numberOfOutliers = numOutliers;
end

== matlab function AVE_Library/Navigation/Sensor Preprocessing/Detect Outliers GNSS/MATLAB Function ==
  data: triggerNewData input boolean size=1; positionLLA input double size=3; numberOfOutliers output uint32 size=1; thresholdHorizontal input double size=1; thresholdVertical input double size=1; maxNumOutliers input uint32 size=1
function numberOfOutliers = DetectOutlier(triggerNewData, positionLLA, thresholdHorizontal, thresholdVertical, maxNumOutliers)
    persistent prevPositionLLA; if(isempty(prevPositionLLA)), prevPositionLLA = positionLLA; end
    persistent numOutliers; if(isempty(numOutliers)), numOutliers = uint32(0); end

    % New data must be available
    if(triggerNewData)
        % Check whether the new data indicates an outlier
        [N, E, D] = ave.LLA2NED(prevPositionLLA(1), prevPositionLLA(2), prevPositionLLA(3), positionLLA(1), positionLLA(2), prevPositionLLA(3));
        horizontalDistance = sqrt(N*N + E*E);
        verticalDistance = abs(D);
        outlier = (horizontalDistance >= abs(thresholdHorizontal)) || (verticalDistance >= abs(thresholdVertical));

        % If it's an outlier, increment the counter
        % If not, save new previous value and reset counter
        if(outlier)
            % If the maximum number of outliers is exceeded, then ignore the outlier and assume it as a valid value
            if(numOutliers >= uint32(maxNumOutliers))
                prevPositionLLA = positionLLA;
                numOutliers = uint32(0);
            else
                numOutliers = numOutliers + uint32(1);
            end
        else
            prevPositionLLA = positionLLA;
            numOutliers = uint32(0);
        end
    end

    % Set output
    numberOfOutliers = numOutliers;
end

== matlab function AVE_Library/Essential/Positive Angle/MATLAB Function ==
  data: u input; y output
function y = PA(u)
    y = ave.PositiveAngle(u);
end

== matlab function AVE_Library/Navigation/Sensor Preprocessing/Detect Outliers Angle 1D/MATLAB Function ==
  data: triggerNewData input boolean size=1; data input double size=1; numberOfOutliers output uint32 size=1; threshold input double size=1; maxNumOutliers input uint32 size=1
function numberOfOutliers = DetectOutlier(triggerNewData, data, threshold, maxNumOutliers)
    persistent prevData; if(isempty(prevData)), prevData = data; end
    persistent numOutliers; if(isempty(numOutliers)), numOutliers = uint32(0); end

    % New data must be available
    if(uint8(triggerNewData))
        % Check whether the new data indicates an outlier
        outlier = abs(ave.SymmetricalAngle(data - prevData)) >= abs(threshold);

        % If it's an outlier, increment the counter
        % If not, save new previous value and reset counter
        if(outlier)
            % If the maximum number of outliers is exceeded, then ignore the outlier and assume it as a valid value
            if(numOutliers >= uint32(maxNumOutliers))
                prevData = data;
                numOutliers = uint32(0);
            else
                numOutliers = numOutliers + uint32(1);
            end
        else
            prevData = data;
            numOutliers = uint32(0);
        end
    end

    % Set output
    numberOfOutliers = numOutliers;
end

== matlab function AVE_Library/Navigation/Sensor Preprocessing/Butterworth Filter/Butterworth Low Pass and Derivation/Subsystem/Butter 2 p,k1 ==
  data: p output; n_Ordnung_Butter_Simulink parameter
function p  = fcn(n_Ordnung_Butter_Simulink)
n=n_Ordnung_Butter_Simulink;



iterator=[1:2:n-1];
n_p1=length(iterator);
p1=zeros(1,n_p1);
p3=zeros(n*n_p1,1);
n = double(n);
% Poles are on the unit circle in the left-half plane.
p1 = exp(1i*(pi*(1:2:n-1)/(2*n) + pi/2));
p2 = [p1; conj(p1)];
p3 = p2(:);
if rem(n,2)==1   % n is odd
    p = [p3; -1];
else
    p=p3;
end
p = cplxpair(p,0);
end
